simulink model "speedgoat_test_SN6848_R2021a"  (R2021a)
settings: Solver=FixedStepDiscrete  StartTime=0.0  StopTime=20  RelTol=1e-3
PreLoadFcn:
  | Ts = 0.001;
  | FPGA_Frequency = 75000000;
  | 
  | Ts = 0.001;
  | FPGA_Frequency = 75000000;
  | 
  | ts_IO691 = 5e-3;
InitFcn:
  | Ts = 0.001;
  | FPGA_Frequency = 75000000;
  | 
  | Ts = 0.001;
  | FPGA_Frequency = 75000000;
  | 
  | ts_IO691 = 5e-3;
StopFcn:
  | Simulink.sdi.clearPreferences;
  | if isfile(['sdi_view_',bdroot,'.mldatx'])
  | Simulink.sdi.view;
  | pause(3);
  | Simulink.sdi.loadView(['sdi_view_',bdroot,]);
  | end
undefined symbols (not defined in the file): IO397
libraries: speedgoatlib_fpga_dio x6, canmsglib x6, speedgoatlib_IO691 x5, speedgoatlib_fpga_analog_io x4, simulink x3, speedgoatlib_fpga_inta x2, speedgoatlib_interrupt x2, speedgoatlib_fpga x2
settings Model: Creator=yannick.orgas  LastModifiedBy=yannick.orgas
settings SolverCC: ConcurrentTasks=on  PositivePriorityOrder=on
settings DataIOCC: LimitDataPoints=on  SaveFormat=StructureWithTime
settings OptimizationCC: BlockReduction=off  OptimizeBlockIOStorage=off
settings DebuggingCC: TasksWithSamePriorityMsg=none  UnconnectedInputMsg=none  UnconnectedOutputMsg=none  UnconnectedLineMsg=none
settings HardwareCC: ProdBitPerLong=64  ProdLongLongMode=on  ProdHWDeviceType=Intel->x86-64 (Linux 64)
settings RTWCC: Description=Simulink Real-Time  SystemTargetFile=slrealtime.tlc  TemplateMakefile=slrealtime_default_tmf  RTWVerbose=off  Toolchain=Simulink Real-Time Toolchain  BuildConfiguration=Faster Runs  CodeExecutionProfiling=on  TargetLang=C++

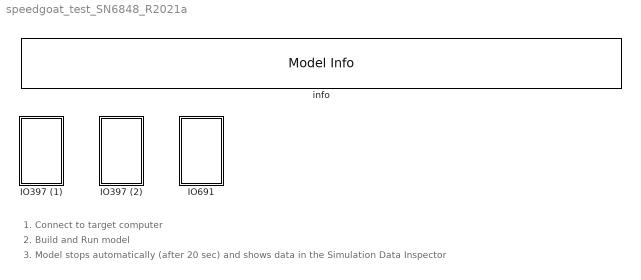
== system speedgoat_test_SN6848_R2021a ==
  note: 1. Connect to target computer
  note: 2. Build and Run model
  note: 3. Model stops automatically (after 20 sec) and shows data in the Simulation Data Inspector
  IO397 (1) : Subsystem
  IO397 (2) : Subsystem
  IO691 : Subsystem
  info : simulink/Model-Wide Utilities/Model Info  Frame=on  DisplayStringWithTags=SPEEDGOAT Simulink Real-Time test model for real-time target machine (SN6848)  HorizontalTextAlignment=Left  LeftAlignmentValue=0.02

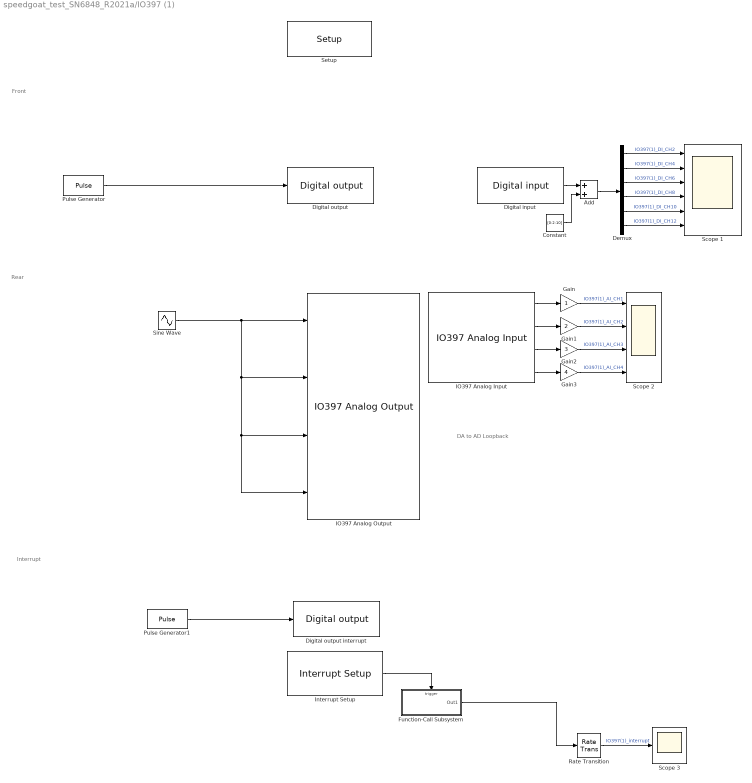
== system speedgoat_test_SN6848_R2021a/IO397 (1) ==
  note: Front
  note: Interrupt
  note: Rear
  note: DA to AD Loopback
  Add : Sum
  Constant : Constant  Value=[0:2:10]
  Demux : Demux  Outputs=6
  Digital input : speedgoatlib_fpga_dio/Digital input  id=1  chan=[2 4 6 8 10 12]  ts=Ts  pciSlot=[6,0]  board=IO397-50k  vectorizeOutput=on
      settings: SourceProductName=Simulink Real-Time: Speedgoat I/O Driver Library
  Digital output : speedgoatlib_fpga_dio/Digital output  id=1  chan=[1 3 5 7 9 11]  init=[0]  reset=[0]  vectorizeInput=on  ts=Ts  pciSlot=[6,0]  board=IO397-50k
      settings: SourceProductName=Simulink Real-Time: Speedgoat I/O Driver Library
  Digital output interrupt : speedgoatlib_fpga_dio/Digital output  id=1  chan=13  init=[0]  reset=[0]  vectorizeInput=on  ts=Ts  pciSlot=[6,0]  board=IO397-50k
      settings: SourceProductName=Simulink Real-Time: Speedgoat I/O Driver Library
  Function-Call Subsystem : Subsystem  TreatAsAtomicUnit=on
  Gain : Gain
  Gain1 : Gain  Gain=2
  Gain2 : Gain  Gain=3
  Gain3 : Gain  Gain=4
  IO397 Analog Input : speedgoatlib_fpga_analog_io/IO397 Analog Input  id=1  chan=[1:4]  range=+-5.12 V  trigger=Initiator  ts=0.001  pciSlot=[6,0]  board=IO397-50k
      settings: SourceProductName=Simulink Real-Time: Speedgoat I/O Driver Library
  IO397 Analog Output : speedgoatlib_fpga_analog_io/IO397 Analog Output  id=1  chan=1:4  initVal=0  resetVal=0  ts=0.001  pciSlot=[6,0]  board=IO397-50k  span=+-5 V
      settings: SourceProductName=Simulink Real-Time: Speedgoat I/O Driver Library
  Interrupt Setup : speedgoatlib_interrupt/Interrupt Setup  parModuleTrigger=off  parPollingMode=off  parPriorityConf=High  parPriority=241  confStartFcn=IO397_50k_start_public  confStopFcn=IO397_50k_stop_public  confIsrFcn=IO397_50k_isr_public  confMapFcn=IO397_50k_map_public  confHookFile=io397_50k_int_hooks.c  confIrqNr=-1  confIsMdlTrig=off  confIsPolling=off  confPriority=254  confModID=1  confSelectedInt=Speedgoat IO397-50k interrupt  confSelectedId=1
  Pulse Generator : DiscretePulseGenerator  Amplitude=ones(1,6)  Period=20  PulseWidth=10  SampleTime=Ts
  Pulse Generator1 : DiscretePulseGenerator  SampleTime=Ts
  Rate Transition : RateTransition  Integrity=off
  Scope 1 : Scope  NumInputPorts=6
  Scope 2 : Scope  NumInputPorts=4
  Scope 3 : Scope
  Setup : speedgoatlib_fpga/Setup/Setup  board=IO397-50k  id=1  device_id=1  frontIO=None  rearIO=None  bitstreamFile=speedgoat_IO397_50k_all_io.mat  rev=1.0  timestamp_string=21/11/18 14:52:53  fpgaFreq=75 MHz  fpgaTick=13.33 ns  ProgSpiFlash=off  ProgBPIFlash=off  pciSlot=[6,0]  PullRPort0=pull-up 3.3V  VioPort0=3.3V  PullRPort1=pull-up 3.3V  VioPort1=3.3V  PullRPort2=pull-up 3.3V  VioPort2=3.3V  PullRPort3=pull-up 3.3V  VioPort3=3.3V  PullRPort4=pull-up 3.3V  VioPort4=3.3V  PullRPort5=pull-up 3.3V  VioPort5=3.3V  PullRPort6=pull-up 3.3V  VioPort6=3.3V  PullRPort15=pull-up 3.3V  PullRPort31=pull-up 3.3V  PullRPort47=pull-up 3.3V  PullRPort63=pull-up 3.3V
      settings: SourceProductName=Simulink Real-Time: Speedgoat I/O Driver Library
  Sine Wave : Sin  Frequency=2*pi*(1/Ts)/50  SampleTime=Ts
  wires:
  Function-Call Subsystem/1(Out1) -> Rate Transition/1
  Digital input/1 -> Add/1
  Pulse Generator1/1 -> Digital output interrupt/1
  Pulse Generator/1 -> Digital output/1
  IO397 Analog Input/4 -> Gain3/1
  IO397 Analog Input/2 -> Gain1/1
  IO397 Analog Input/3 -> Gain2/1
  IO397 Analog Input/1 -> Gain/1
  Sine Wave/1 -> IO397 Analog Output/1, IO397 Analog Output/4, IO397 Analog Output/3, IO397 Analog Output/2
  Constant/1 -> Add/2
  Gain/1 -> Scope 2/1  "IO397(1)_AI_CH1"
  Gain1/1 -> Scope 2/2  "IO397(1)_AI_CH2"
  Gain2/1 -> Scope 2/3  "IO397(1)_AI_CH3"
  Gain3/1 -> Scope 2/4  "IO397(1)_AI_CH4"
  Rate Transition/1 -> Scope 3/1  "IO397(1)_interrupt"
  Interrupt Setup/1 -> Function-Call Subsystem/Trigger
  Add/1 -> Demux/1
  Demux/1 -> Scope 1/1  "IO397(1)_DI_CH2"
  Demux/2 -> Scope 1/2  "IO397(1)_DI_CH4"
  Demux/3 -> Scope 1/3  "IO397(1)_DI_CH6"
  Demux/4 -> Scope 1/4  "IO397(1)_DI_CH8"
  Demux/5 -> Scope 1/5  "IO397(1)_DI_CH10"
  Demux/6 -> Scope 1/6  "IO397(1)_DI_CH12"

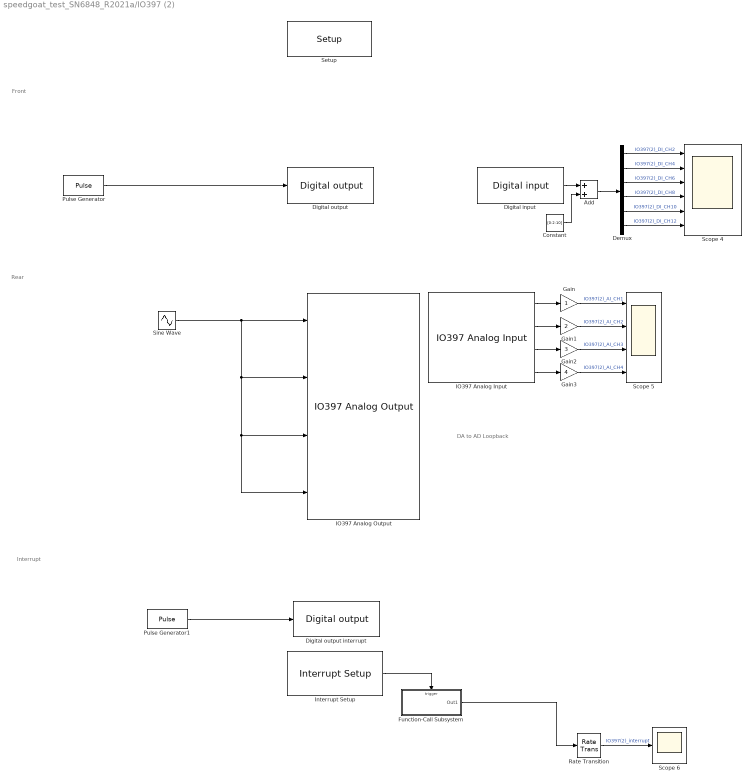
== system speedgoat_test_SN6848_R2021a/IO397 (2) ==
  note: Front
  note: Interrupt
  note: Rear
  note: DA to AD Loopback
  Add : Sum
  Constant : Constant  Value=[0:2:10]
  Demux : Demux  Outputs=6
  Digital input : speedgoatlib_fpga_dio/Digital input  id=2  chan=[2 4 6 8 10 12]  ts=Ts  pciSlot=[11,0]  board=IO397-50k  vectorizeOutput=on
      settings: SourceProductName=Simulink Real-Time: Speedgoat I/O Driver Library
  Digital output : speedgoatlib_fpga_dio/Digital output  id=2  chan=[1 3 5 7 9 11]  init=[0]  reset=[0]  vectorizeInput=on  ts=Ts  pciSlot=[11,0]  board=IO397-50k
      settings: SourceProductName=Simulink Real-Time: Speedgoat I/O Driver Library
  Digital output interrupt : speedgoatlib_fpga_dio/Digital output  id=2  chan=13  init=[0]  reset=[0]  vectorizeInput=on  ts=Ts  pciSlot=[11,0]  board=IO397-50k
      settings: SourceProductName=Simulink Real-Time: Speedgoat I/O Driver Library
  Function-Call Subsystem : Subsystem  TreatAsAtomicUnit=on
  Gain : Gain
  Gain1 : Gain  Gain=2
  Gain2 : Gain  Gain=3
  Gain3 : Gain  Gain=4
  IO397 Analog Input : speedgoatlib_fpga_analog_io/IO397 Analog Input  id=2  chan=[1:4]  range=+-5.12 V  trigger=Initiator  ts=0.001  pciSlot=[11,0]  board=IO397-50k
      settings: SourceProductName=Simulink Real-Time: Speedgoat I/O Driver Library
  IO397 Analog Output : speedgoatlib_fpga_analog_io/IO397 Analog Output  id=2  chan=1:4  initVal=0  resetVal=0  ts=0.001  pciSlot=[11,0]  board=IO397-50k  span=+-5 V
      settings: SourceProductName=Simulink Real-Time: Speedgoat I/O Driver Library
  Interrupt Setup : speedgoatlib_interrupt/Interrupt Setup  parModuleTrigger=off  parPollingMode=off  parPriorityConf=High  parPriority=241  confStartFcn=IO397_50k_start_public  confStopFcn=IO397_50k_stop_public  confIsrFcn=IO397_50k_isr_public  confMapFcn=IO397_50k_map_public  confHookFile=io397_50k_int_hooks.c  confIrqNr=-1  confIsMdlTrig=off  confIsPolling=off  confPriority=254  confModID=2  confSelectedInt=Speedgoat IO397-50k interrupt  confSelectedId=2
  Pulse Generator : DiscretePulseGenerator  Amplitude=ones(1,6)  Period=20  PulseWidth=10  SampleTime=Ts
  Pulse Generator1 : DiscretePulseGenerator  SampleTime=Ts
  Rate Transition : RateTransition  Integrity=off
  Scope 4 : Scope  NumInputPorts=6
  Scope 5 : Scope  NumInputPorts=4
  Scope 6 : Scope
  Setup : speedgoatlib_fpga/Setup/Setup  board=IO397-50k  id=2  device_id=2  frontIO=None  rearIO=None  bitstreamFile=speedgoat_IO397_50k_all_io.mat  rev=1.0  timestamp_string=21/11/18 14:52:53  fpgaFreq=75 MHz  fpgaTick=13.33 ns  ProgSpiFlash=off  ProgBPIFlash=off  pciSlot=[11,0]  PullRPort0=pull-up 3.3V  VioPort0=3.3V  PullRPort1=pull-up 3.3V  VioPort1=3.3V  PullRPort2=pull-up 3.3V  VioPort2=3.3V  PullRPort3=pull-up 3.3V  VioPort3=3.3V  PullRPort4=pull-up 3.3V  VioPort4=3.3V  PullRPort5=pull-up 3.3V  VioPort5=3.3V  PullRPort6=pull-up 3.3V  VioPort6=3.3V  PullRPort15=pull-up 3.3V  PullRPort31=pull-up 3.3V  PullRPort47=pull-up 3.3V  PullRPort63=pull-up 3.3V
      settings: SourceProductName=Simulink Real-Time: Speedgoat I/O Driver Library
  Sine Wave : Sin  Frequency=2*pi*(1/Ts)/50  SampleTime=Ts
  wires:
  Function-Call Subsystem/1(Out1) -> Rate Transition/1
  Digital input/1 -> Add/1
  Pulse Generator1/1 -> Digital output interrupt/1
  Pulse Generator/1 -> Digital output/1
  IO397 Analog Input/4 -> Gain3/1
  IO397 Analog Input/2 -> Gain1/1
  IO397 Analog Input/3 -> Gain2/1
  IO397 Analog Input/1 -> Gain/1
  Sine Wave/1 -> IO397 Analog Output/1, IO397 Analog Output/4, IO397 Analog Output/3, IO397 Analog Output/2
  Constant/1 -> Add/2
  Gain/1 -> Scope 5/1  "IO397(2)_AI_CH1"
  Gain1/1 -> Scope 5/2  "IO397(2)_AI_CH2"
  Gain2/1 -> Scope 5/3  "IO397(2)_AI_CH3"
  Gain3/1 -> Scope 5/4  "IO397(2)_AI_CH4"
  Rate Transition/1 -> Scope 6/1  "IO397(2)_interrupt"
  Interrupt Setup/1 -> Function-Call Subsystem/Trigger
  Add/1 -> Demux/1
  Demux/1 -> Scope 4/1  "IO397(2)_DI_CH2"
  Demux/2 -> Scope 4/2  "IO397(2)_DI_CH4"
  Demux/3 -> Scope 4/3  "IO397(2)_DI_CH6"
  Demux/4 -> Scope 4/4  "IO397(2)_DI_CH8"
  Demux/5 -> Scope 4/5  "IO397(2)_DI_CH10"
  Demux/6 -> Scope 4/6  "IO397(2)_DI_CH12"

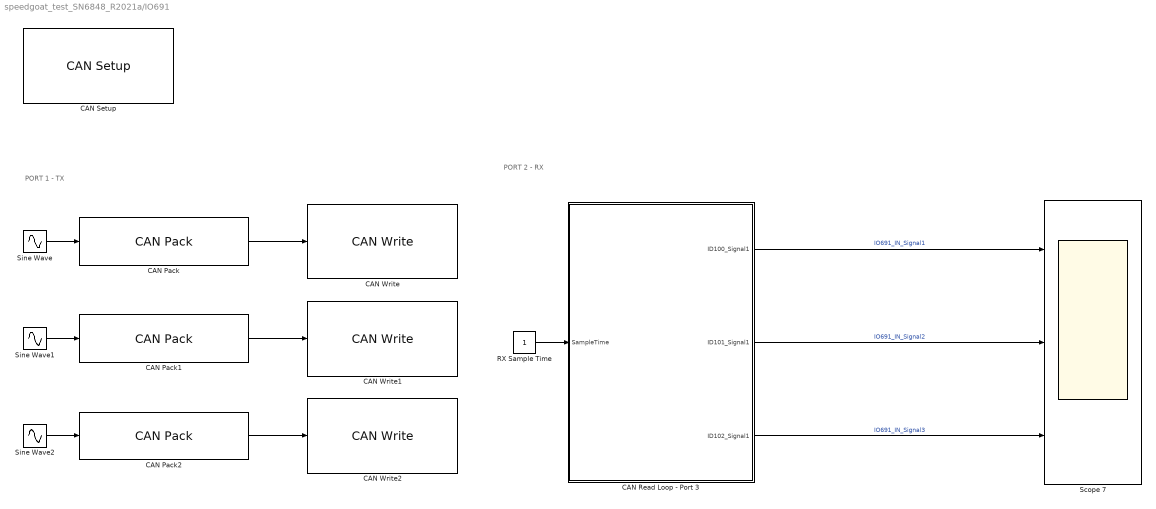
== system speedgoat_test_SN6848_R2021a/IO691 ==
  note: PORT 1 - TX
  note: PORT 2 - RX
  CAN Pack : canmsglib/CAN Pack  MsgList=(none)  MsgName=CAN Msg  MsgIDType=Standard (11-bit identifier)  MsgIdentifier=100  MsgLength=8  Remote=off  ApplyMinMax=off  BusOutput=off  SignalInfo={'Signal1','0','64','LE','double','Standard','0','1','0','-Inf','Inf'}
      settings: SourceProductBaseCode=ME,XP,VN  DataFormat=manually specified signals
  CAN Pack1 : canmsglib/CAN Pack  MsgList=(none)  MsgName=CAN Msg  MsgIDType=Standard (11-bit identifier)  MsgIdentifier=101  MsgLength=8  Remote=off  ApplyMinMax=off  BusOutput=off  SignalInfo={'Signal1','0','64','LE','double','Standard','0','1','0','-Inf','Inf'}
      settings: SourceProductBaseCode=ME,XP,VN  DataFormat=manually specified signals
  CAN Pack2 : canmsglib/CAN Pack  MsgList=(none)  MsgName=CAN Msg  MsgIDType=Standard (11-bit identifier)  MsgIdentifier=102  MsgLength=8  Remote=off  ApplyMinMax=off  BusOutput=off  SignalInfo={'Signal1','0','64','LE','double','Standard','0','1','0','-Inf','Inf'}
      settings: SourceProductBaseCode=ME,XP,VN  DataFormat=manually specified signals
  CAN Read Loop - Port 3 : Subsystem  TreatAsAtomicUnit=on
  "CAN Setup " : speedgoatlib_IO691/CAN Setup   moduletype=IO691  id=1  pciSlot=-1  chn1=CAN (HS)  chn2=CAN (HS)  chn3=Disabled  chn4=Disabled  initStruct=[]  termStruct=[]  ArbitrationbdrChn1=1.0 MBaud  ArbitrationManbdrChn1=[2,8,31,8]  FdbdrChn1=5.0 MBaud  FdManbdrChn1=[2,2,5,2]  ArbitrationbdrChn2=1.0 MBaud  ArbitrationManbdrChn2=[2,8,31,8]  FdbdrChn2=5.0 MBaud  FdManbdrChn2=[2,2,5,2]  ArbitrationbdrChn3=1.0 MBaud  ArbitrationManbdrChn3=[2,8,31,8]  FdbdrChn3=5.0 MBaud  FdManbdrChn3=[2,2,5,2]  ArbitrationbdrChn4=1.0 MBaud  ArbitrationManbdrChn4=[2,8,31,8]  FdbdrChn4=5.0 MBaud  FdManbdrChn4=[2,2,5,2]  moduleInitValues=[691 1 -1 -1]
      settings: SourceProductName=Simulink Real-Time: Speedgoat Library
  CAN Write : speedgoatlib_IO691/CAN Write  id=1  ts=-1  channel=1  messageType=CAN  enableStatusPort=off  canType=CAN (HS)  initValues=[691 1 -1 0 1 1 0]
      settings: SourceProductName=Simulink Real-Time: Speedgoat Library
  CAN Write1 : speedgoatlib_IO691/CAN Write  id=1  ts=-1  channel=1  messageType=CAN  enableStatusPort=off  canType=CAN (HS)  initValues=[691 1 -1 0 1 1 0]
      settings: SourceProductName=Simulink Real-Time: Speedgoat Library
  CAN Write2 : speedgoatlib_IO691/CAN Write  id=1  ts=-1  channel=1  messageType=CAN  enableStatusPort=off  canType=CAN (HS)  initValues=[691 1 -1 0 1 1 0]
      settings: SourceProductName=Simulink Real-Time: Speedgoat Library
  RX Sample Time : Constant  SampleTime=ts_IO691
  Scope 7 : Scope  NumInputPorts=3
  Sine Wave : Sin  Amplitude=10  Frequency=2*pi*10  SampleTime=ts_IO691
  Sine Wave1 : Sin  Amplitude=20  Frequency=2*pi*10  SampleTime=ts_IO691
  Sine Wave2 : Sin  Amplitude=30  Frequency=2*pi*10  SampleTime=ts_IO691
  wires:
  RX Sample Time/1 -> CAN Read Loop - Port 3/1(SampleTime)
  Sine Wave1/1 -> CAN Pack1/1
  Sine Wave/1 -> CAN Pack/1
  Sine Wave2/1 -> CAN Pack2/1
  CAN Pack/1 -> CAN Write/1
  CAN Pack1/1 -> CAN Write1/1
  CAN Pack2/1 -> CAN Write2/1
  CAN Read Loop - Port 3/1(ID100_Signal1) -> Scope 7/1  "IO691_IN_Signal1"
  CAN Read Loop - Port 3/2(ID101_Signal1) -> Scope 7/2  "IO691_IN_Signal2"
  CAN Read Loop - Port 3/3(ID102_Signal1) -> Scope 7/3  "IO691_IN_Signal3"

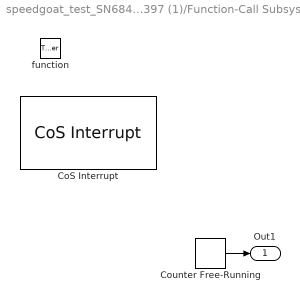
== system speedgoat_test_SN6848_R2021a/IO397 (1)/Function-Call Subsystem ==
  function : TriggerPort  TriggerType=function-call  VariantControl=Variant
  CoS Interrupt : speedgoatlib_fpga_inta/CoS Interrupt  id=1  debounce=0  delay=0  polarity=1  pciSlot=[6,0]  ts=-1  board=IO397-50k
      settings: SourceProductName=Simulink Real-Time: Speedgoat I/O Driver Library
  Counter Free-Running : simulink/Sources/Counter Free-Running  NumBits=32  tsamp=-1
  Out1 : Outport  InitialOutput=[0]
  wires:
  Counter Free-Running/1 -> Out1/1

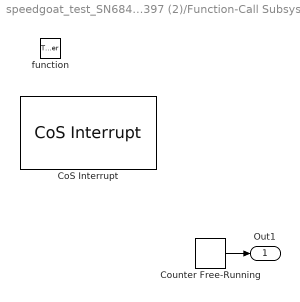
== system speedgoat_test_SN6848_R2021a/IO397 (2)/Function-Call Subsystem ==
  function : TriggerPort  TriggerType=function-call  VariantControl=Variant
  CoS Interrupt : speedgoatlib_fpga_inta/CoS Interrupt  id=2  debounce=0  delay=0  polarity=1  pciSlot=[11,0]  ts=-1  board=IO397-50k
      settings: SourceProductName=Simulink Real-Time: Speedgoat I/O Driver Library
  Counter Free-Running : simulink/Sources/Counter Free-Running  NumBits=32  tsamp=-1
  Out1 : Outport  InitialOutput=[0]
  wires:
  Counter Free-Running/1 -> Out1/1

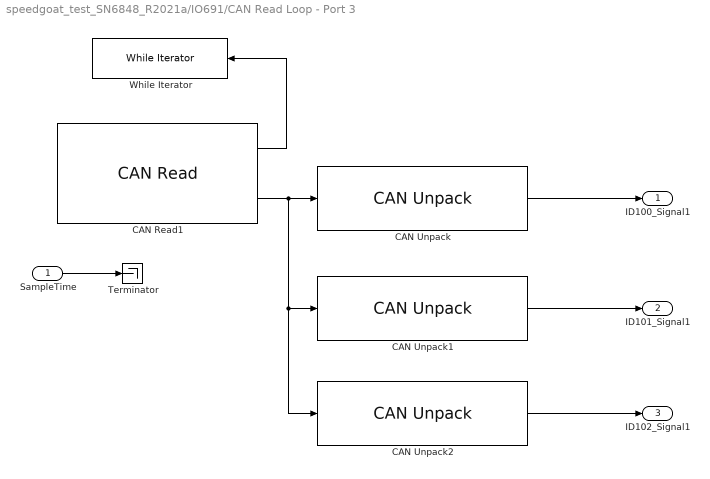
== system speedgoat_test_SN6848_R2021a/IO691/CAN Read Loop - Port 3 ==
  SampleTime : Inport
  CAN Read1 : speedgoatlib_IO691/CAN Read  id=1  ts=-1  channel=2  messageType=CAN  canType=CAN (HS)  initValues=[691 1 -1 1 1 1]
      settings: SourceProductName=Simulink Real-Time: Speedgoat Library
  CAN Unpack : canmsglib/CAN Unpack  MsgList=(none)  MsgName=CAN Msg  MsgIDType=Standard (11-bit identifier)  MsgIdentifier=100  MsgLength=8  SignalInfo={'Signal1','0','64','LE','double','Standard','0','1','0','-Inf','Inf'}  IDPort=off  TimestampPort=off  ErrorPort=off  RemotePort=off  LengthPort=off  StatusPort=off  ApplyMinMax=off
      settings: SourceProductBaseCode=ME,XP,VN
  CAN Unpack1 : canmsglib/CAN Unpack  MsgList=(none)  MsgName=CAN Msg  MsgIDType=Standard (11-bit identifier)  MsgIdentifier=101  MsgLength=8  SignalInfo={'Signal1','0','64','LE','double','Standard','0','1','0','-Inf','Inf'}  IDPort=off  TimestampPort=off  ErrorPort=off  RemotePort=off  LengthPort=off  StatusPort=off  ApplyMinMax=off
      settings: SourceProductBaseCode=ME,XP,VN
  CAN Unpack2 : canmsglib/CAN Unpack  MsgList=(none)  MsgName=CAN Msg  MsgIDType=Standard (11-bit identifier)  MsgIdentifier=102  MsgLength=8  SignalInfo={'Signal1','0','64','LE','double','Standard','0','1','0','-Inf','Inf'}  IDPort=off  TimestampPort=off  ErrorPort=off  RemotePort=off  LengthPort=off  StatusPort=off  ApplyMinMax=off
      settings: SourceProductBaseCode=ME,XP,VN
  Terminator : Terminator
  While Iterator : WhileIterator  MaxIters=501  WhileBlockType=do-while
  ID100_Signal1 : Outport
  ID101_Signal1 : Outport  Port=2
  ID102_Signal1 : Outport  Port=3
  wires:
  SampleTime/1 -> Terminator/1
  CAN Unpack2/1 -> ID102_Signal1/1
  CAN Unpack1/1 -> ID101_Signal1/1
  CAN Unpack/1 -> ID100_Signal1/1
  CAN Read1/1 -> While Iterator/1
  CAN Read1/2 -> CAN Unpack/1, CAN Unpack1/1, CAN Unpack2/1
